simulink model "Test_TCPSocket_Client"  (R2019a)
settings: Solver=FixedStepDiscrete  StartTime=0.0  StopTime=10  RelTol=1e-6  AbsTol=1e-6  EnableMultiTasking=on
InitFcn:
  | clear('all');
settings Model: Creator=Andreas Schellenberg  LastModifiedBy=Andreas
settings SolverCC: AutoScaleAbsTol=off
settings DataIOCC: SaveFormat=StructureWithTime  SignalLoggingSaveFormat=ModelDataLogs  SaveState=on  SignalLogging=off  ReturnWorkspaceOutputs=off  SignalLoggingName=sigsOut  OutputOption=SpecifiedOutputTimes  OutputTimes=t
settings OptimizationCC: ExpressionDepthLimit=2147483647  InitFltsAndDblsToZero=on  LifeSpan=inf
settings DebuggingCC: SaveWithParameterizedLinksMsg=none  UnderspecifiedInitializationDetection=Classic  MergeDetectMultiDrivingBlocksExec=none  SignalResolutionControl=TryResolveAllWithWarning  MultiTaskDSMMsg=warning  MultiTaskCondExecSysMsg=none  FcnCallInpInsideContextMsg=warning  StateNameClashWarn=warning  SFUnexpectedBacktrackingDiag=warning  SFNoUnconditionalDefaultTransitionDiag=warning  SFExecutionAtInitializationDiag=none  ArithmeticOperatorsInVariantConditions=warning
settings HardwareCC: ProdBitPerPointer=32  ProdBitPerSizeT=32  ProdBitPerPtrDiffT=32  ProdLargestAtomicFloat=None  ProdIntDivRoundTo=Undefined  ProdEndianess=Unspecified  ProdWordSize=32  ProdHWDeviceType=32-bit Generic  TargetUnknown=on
settings ModelReferenceCC: PropagateSignalLabelsOutOfModel=off
settings SFSimCC: SimUseLocalCustomCode=off
settings RTWCC: RTWUseLocalCustomCode=off
settings CodeAppCC: StateflowObjectComments=on
settings GRTTargetCC: TargetLangStandard=C89/C90 (ANSI)  CombineOutputUpdateFcns=off  GRTInterface=on
settings ConfigComp: CovMetricSettings=dw  CovHtmlReporting=on  CovSaveCumulativeToWorkspaceVar=on  CovSaveSingleToWorkspaceVar=on

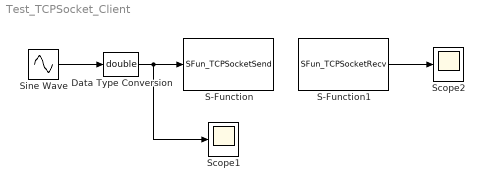
== system Test_TCPSocket_Client ==
  Data Type Conversion : DataTypeConversion  OutDataTypeStr=double
  S-Function : S-Function  FunctionName=SFun_TCPSocketSend  Parameters=ipAddr,ipPort  SFunctionDeploymentMode=off  EnableBusSupport=off  mask(TCP Socket Send){ipAddr=127.0.0.1, ipPort=8090}
      mask prompts: ipAddr "IP Address of Server (leave empty if defining a Server)"; ipPort "IP Port Number of Server or Client"
      mask Display: disp('TCP Socket\nSend');
  S-Function1 : S-Function  FunctionName=SFun_TCPSocketRecv  Parameters=ipAddr,ipPort,dataType,sampleTime  SFunctionDeploymentMode=off  EnableBusSupport=off  mask(TCP Socket Receive){ipAddr=127.0.0.1, ipPort=8091, dataType=double, sampleTime=0.01}
      mask prompts: ipAddr "IP Address of Server (leave empty if defining a Server)"; ipPort "IP Port Number of Server or Client"; dataType "Data Type"; sampleTime "Sample Time"
      mask TypeOptions dataType: double | single | int32 | int16 | int8
      mask Display: disp('TCP Socket\nReceive');
  Scope1 : Scope
  Scope2 : Scope
  Sine Wave : Sin  Amplitude=10  Frequency=pi  SampleTime=0.01
  wires:
  Sine Wave/1 -> Data Type Conversion/1
  S-Function1/1 -> Scope2/1
  Data Type Conversion/1 -> S-Function/1, Scope1/1
